simulink model "series_link_blance_leg1"  (R2022b)
settings: Solver=ode45  StartTime=0.0  StopTime=20  MaxStep=0.2  RelTol=1e-3
values from neighbouring files (symbols this model uses):
  a11 = polyfit(leg,k11,2)    [series_get_k.m]
  a12 = polyfit(leg,k12,2)    [series_get_k.m]
  a13 = polyfit(leg,k13,1)    [series_get_k.m]
  a14 = polyfit(leg,k14,2)    [series_get_k.m]
  N = mp*diff(x + L*sin(theta),t,2)    [series_get_k1_length.m]
undefined symbols (not defined in the file or in its folder): X, Y, Z
libraries: sm_lib x59, nesl_utility x10, slpidlib x2, matrix_library x2
(part 3 of 3)

== matlab function series_link_blance_leg1/control1/MATLAB Function6 ==
  data: F0 input; T_joint output; theta1 input
function T_joint = VMC_calc(F0,theta1)
    l1 = 0.163; %%163.04mm
    l2 = 0.165; %%164.75mm
    l3 = 0.170; %%170.15mm
    l4 = 0.08;  %%79.5mm
    l23 = 0.04;  %%40.05mm

    J = l2*cos(theta1) + l1*cos(theta1 + acos((l2^2 - 2*cos(pi/4 + theta1)*l2*l4 - l3^2 + l4^2 + l23^2)/(2*l23*(l2^2 - 2*cos(pi/4 + theta1)*l2*l4 + l4^2)^(1/2))) + asin((l4*sin(theta1 + pi/4))/(l2^2 - 2*cos(pi/4 + theta1)*l2*l4 + l4^2)^(1/2)))*(((l4*cos(theta1 + pi/4))/(l2^2 - 2*cos(pi/4 + theta1)*l2*l4 + l4^2)^(1/2) - (l2*l4^2*sin(theta1 + pi/4)^2)/(l2^2 - 2*cos(pi/4 + theta1)*l2*l4 + l4^2)^(3/2))/(1 - (l4^2*sin(theta1 + pi/4)^2)/(l2^2 - 2*cos(pi/4 + theta1)*l2*l4 + l4^2))^(1/2) - ((l2*l4*sin(theta1 + pi/4))/(l23*(l2^2 - 2*cos(pi/4 + theta1)*l2*l4 + l4^2)^(1/2)) - (l2*l4*sin(theta1 + pi/4)*(l2^2 - 2*cos(pi/4 + theta1)*l2*l4 - l3^2 + l4^2 + l23^2))/(2*l23*(l2^2 - 2*cos(pi/4 + theta1)*l2*l4 + l4^2)^(3/2)))/(1 - (l2^2 - 2*cos(pi/4 + theta1)*l2*l4 - l3^2 + l4^2 + l23^2)^2/(4*l23^2*(l2^2 - 2*cos(pi/4 + theta1)*l2*l4 + l4^2)))^(1/2) + 1);
    T_joint = F0*J;

end

== matlab function series_link_blance_leg1/control1/MATLAB Function7 ==
  data: L0 output; theta1 input
function L0 = L0(theta1)
    l1 = 0.163; %%163.04mm
    l2 = 0.165; %%164.75mm
    l3 = 0.170; %%170.15mm
    l4 = 0.08;  %%79.5mm
    l23 = 0.04;  %%40.05mm

    
    l5 = sqrt(l2^2 + l4^2 -2*l2*l4*cos(theta1 + pi/4));
    theta2 = asin(l4*sin(theta1 + pi/4)/l5);
    theta3 = acos((l23^2+l5^2-l3^2)/(2*l23*l5));
    theta4 =theta1 + theta2 +theta3;
    yc = l2*sin(theta1) + l1*sin(theta4);
    L0 = yc;

end

== matlab function series_link_blance_leg1/calc/MATLAB Function6 ==
  data: k output; a input; length input
function k = get_K(a,length)
   k = polyval(a,length);  
end

== matlab function series_link_blance_leg1/calc/MATLAB Function1 ==
  data: k output; a input; length input
function k = get_K(a,length)
   k = polyval(a,length);  
end

== matlab function series_link_blance_leg1/calc/MATLAB Function2 ==
  data: k output; a input; length input
function k = get_K(a,length)
   k = polyval(a,length);  
end

== matlab function series_link_blance_leg1/calc/MATLAB Function3 ==
  data: k output; a input; length input
function k = get_K(a,length)
   k = polyval(a,length);  
end

== matlab function series_link_blance_leg1/calc1/MATLAB Function1 ==
  data: k output; a input; length input
function k = get_K(a,length)
   k = polyval(a,length);  
end

== matlab function series_link_blance_leg1/calc1/MATLAB Function2 ==
  data: k output; a input; length input
function k = get_K(a,length)
   k = polyval(a,length);  
end

== matlab function series_link_blance_leg1/control/MATLAB Function6 ==
  data: F0 input; T_joint output; theta1 input
function T_joint = VMC_calc(F0,theta1)
    l1 = 0.163; %%163.04mm
    l2 = 0.165; %%164.75mm
    l3 = 0.170; %%170.15mm
    l4 = 0.08;  %%79.5mm
    l23 = 0.04;  %%40.05mm

    J = l2*cos(theta1) + l1*cos(theta1 + acos((l2^2 - 2*cos(pi/4 + theta1)*l2*l4 - l3^2 + l4^2 + l23^2)/(2*l23*(l2^2 - 2*cos(pi/4 + theta1)*l2*l4 + l4^2)^(1/2))) + asin((l4*sin(theta1 + pi/4))/(l2^2 - 2*cos(pi/4 + theta1)*l2*l4 + l4^2)^(1/2)))*(((l4*cos(theta1 + pi/4))/(l2^2 - 2*cos(pi/4 + theta1)*l2*l4 + l4^2)^(1/2) - (l2*l4^2*sin(theta1 + pi/4)^2)/(l2^2 - 2*cos(pi/4 + theta1)*l2*l4 + l4^2)^(3/2))/(1 - (l4^2*sin(theta1 + pi/4)^2)/(l2^2 - 2*cos(pi/4 + theta1)*l2*l4 + l4^2))^(1/2) - ((l2*l4*sin(theta1 + pi/4))/(l23*(l2^2 - 2*cos(pi/4 + theta1)*l2*l4 + l4^2)^(1/2)) - (l2*l4*sin(theta1 + pi/4)*(l2^2 - 2*cos(pi/4 + theta1)*l2*l4 - l3^2 + l4^2 + l23^2))/(2*l23*(l2^2 - 2*cos(pi/4 + theta1)*l2*l4 + l4^2)^(3/2)))/(1 - (l2^2 - 2*cos(pi/4 + theta1)*l2*l4 - l3^2 + l4^2 + l23^2)^2/(4*l23^2*(l2^2 - 2*cos(pi/4 + theta1)*l2*l4 + l4^2)))^(1/2) + 1);
    T_joint = F0*J;

end

== matlab function series_link_blance_leg1/control/MATLAB Function7 ==
  data: L0 output; theta1 input
function L0 = L0(theta1)
    l1 = 0.163; %%163.04mm
    l2 = 0.165; %%164.75mm
    l3 = 0.170; %%170.15mm
    l4 = 0.08;  %%79.5mm
    l23 = 0.04;  %%40.05mm

    
    l5 = sqrt(l2^2 + l4^2 -2*l2*l4*cos(theta1 + pi/4));
    theta2 = asin(l4*sin(theta1 + pi/4)/l5);
    theta3 = acos((l23^2+l5^2-l3^2)/(2*l23*l5));
    theta4 =theta1 + theta2 +theta3;
    yc = l2*sin(theta1) + l1*sin(theta4);
    L0 = yc;

end

== matlab function series_link_blance_leg1/calc1/MATLAB Function3 ==
  data: k output; a input; length input
function k = get_K(a,length)
   k = polyval(a,length);  
end

== matlab function series_link_blance_leg1/calc1/MATLAB Function6 ==
  data: k output; a input; length input
function k = get_K(a,length)
   k = polyval(a,length);  
end
